simulink model "zad2model1"  (R2023a)
settings: Solver=VariableStepAuto  StartTime=0.0  StopTime=30  RelTol=1e-3
values from neighbouring files (symbols this model uses):
  Gz = c2d(Gs,T,'zoh')    [zad1.m]
  T = 0.5    [zad1.m]    (also in zad4.mat)
settings Model: Creator=pkutyl  LastModifiedBy=pkutyl

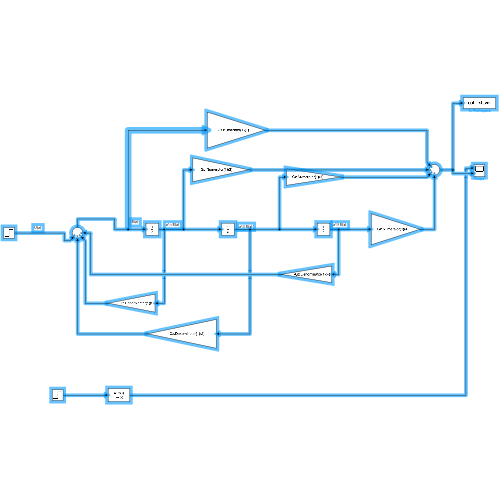
[thumbnail: Simulink's stored preview of the top-level diagram]
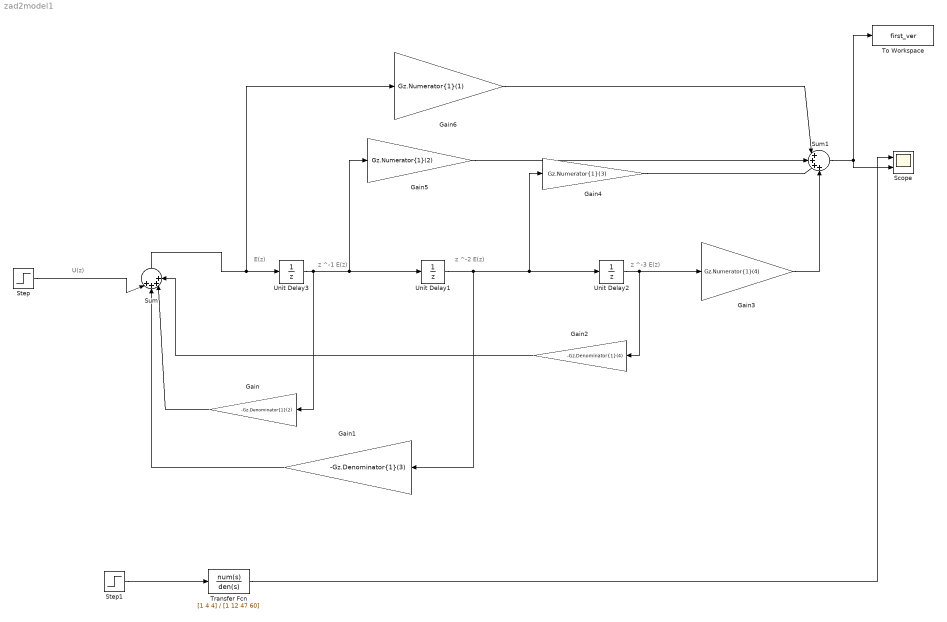
== system zad2model1 ==
  note: U(z)
  note: z ^-1 E(z)
  note: E(z)
  note: z ^-2 E(z)
  note: z ^-3 E(z)
  Gain : Gain  Gain=-Gz.Denominator{1}(2)
  Gain1 : Gain  Gain=-Gz.Denominator{1}(3)
  Gain2 : Gain  Gain=-Gz.Denominator{1}(4)
  Gain3 : Gain  Gain=Gz.Numerator{1}(4)
  Gain4 : Gain  Gain=Gz.Numerator{1}(3)
  Gain5 : Gain  Gain=Gz.Numerator{1}(2)
  Gain6 : Gain  Gain=Gz.Numerator{1}(1)
  Scope : Scope  NumInputPorts=2
  Step : Step  Time=0
  Step1 : Step  Time=0
  Sum : Sum  Inputs=|++++
  Sum1 : Sum  Inputs=|++++
  To Workspace : ToWorkspace  VariableName=first_ver  SaveFormat=Structure With Time  SampleTime=-1
  Transfer Fcn : TransferFcn  Numerator=[1 4 4]  Denominator=[1 12 47 60]
  Unit Delay1 : UnitDelay  SampleTime=T  HasFrameUpgradeWarning=on
  Unit Delay2 : UnitDelay  SampleTime=T  HasFrameUpgradeWarning=on
  Unit Delay3 : UnitDelay  SampleTime=T  HasFrameUpgradeWarning=on
  wires:
  Unit Delay3/1 -> Gain/1, Gain5/1, Unit Delay1/1
  Unit Delay1/1 -> Gain1/1, Gain4/1, Unit Delay2/1
  Sum/1 -> Unit Delay3/1, Gain6/1
  Step/1 -> Sum/1
  Unit Delay2/1 -> Gain2/1, Gain3/1
  Gain1/1 -> Sum/2
  Gain/1 -> Sum/3
  Gain2/1 -> Sum/4
  Gain3/1 -> Sum1/4
  Gain4/1 -> Sum1/3
  Gain5/1 -> Sum1/2
  Sum1/1 -> To Workspace/1, Scope/2
  Gain6/1 -> Sum1/1
  Step1/1 -> Transfer Fcn/1
  Transfer Fcn/1 -> Scope/1
